simulink model "PMSM_EKF"  (R2014b)
settings: Solver=ode23tb  StartTime=0.0  StopTime=0.4  FixedStep=1e-6  RelTol=1e-4
libraries: powerlib x5, powerlib_extras x3, simulink x1
settings Model: Creator=guojinbo  LastModifiedBy=Lei
settings DataIOCC: SignalLoggingSaveFormat=ModelDataLogs
settings OptimizationCC: ExpressionDepthLimit=2147483647  InitFltsAndDblsToZero=on
settings DebuggingCC: UnderspecifiedInitializationDetection=Classic  MergeDetectMultiDrivingBlocksExec=none  FcnCallInpInsideContextMsg=UseLocalSettings  StateNameClashWarn=warning
settings GRTTargetCC: CombineOutputUpdateFcns=off  GRTInterface=on

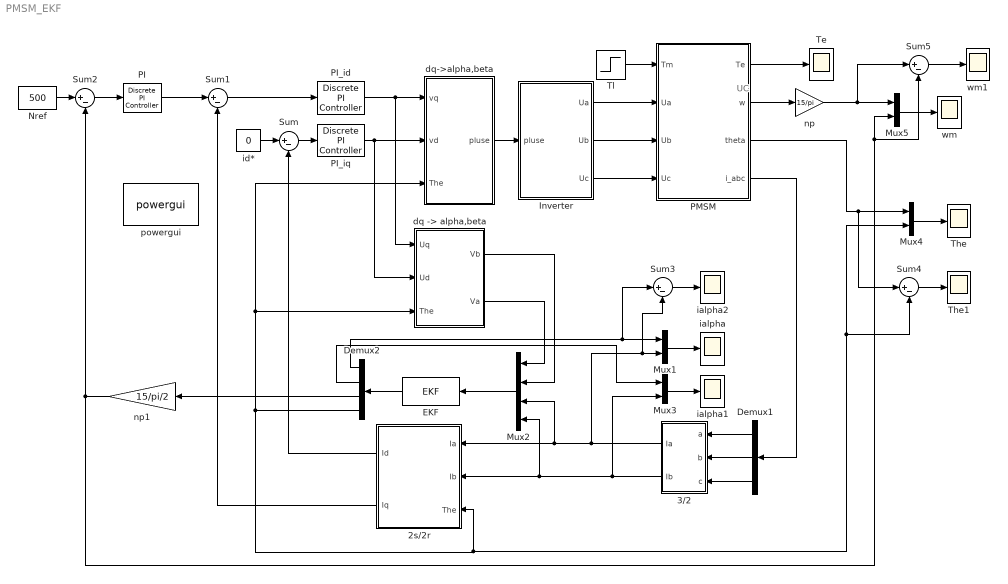
== system PMSM_EKF ==
  note: UC
  " PI " : powerlib_extras/Discrete  Control Blocks/Discrete PI Controller  Kp=0.6  Ki=0.8  Par_Limits=[40 -40]  Init=0  Ts=50e-6
  2s/2r : MATLAB Function  TreatAsAtomicUnit=on
  3/2 : MATLAB Function  TreatAsAtomicUnit=on
  Demux1 : Demux  Outputs=3
  Demux2 : Demux
  EKF : S-Function  FunctionName=EKF  EnableBusSupport=off
  Inverter : Subsystem
  Mux{1,3..5} (4 alike) : Mux  Inputs=2
  Mux2 : Mux
  Nref : Constant  Value=500
  PI_id : powerlib_extras/Discrete  Control Blocks/Discrete PI Controller  Kp=4.8  Ki=5.6  Par_Limits=[200 -200]  Init=0  Ts=50e-6
  PI_iq : powerlib_extras/Discrete  Control Blocks/Discrete PI Controller  Kp=8  Ki=9  Par_Limits=[200 -200]  Init=0  Ts=50e-6
  PMSM : Subsystem
  Sum{,1..5} (6 alike) : Sum  Inputs=|+-
  Te : Scope
      settings: YMin=486  YMax=500  SaveName=Te
  The : Scope
      settings: YMax=25  SaveName=The
  The1 : Scope
      settings: YMin=-0.5  YMax=1  SaveName=Thee
  Tl : Step  Time=0  Before=0.5  After=3.75  SampleTime=0
  "dq -> alpha,beta" : MATLAB Function  TreatAsAtomicUnit=on
  dq->alpha,beta : Subsystem
  ialpha : Scope
      settings: YMin=-100  YMax=600  SaveName=ialpha
  ialpha1 : Scope
      settings: YMin=-100  YMax=600  SaveName=ialpha1
  ialpha2 : Scope
      settings: YMin=-100  YMax=600  SaveName=ialpha2
  id* : Constant  Value=0
  np : Gain  Gain=15/pi
  np1 : Gain  Gain=15/pi/2
  powergui : powerlib/powergui  Priority=2  SimulationMode=Continuous  SolverType=Tustin/Backward Euler (TBE)  SampleTime=50e-6  frequency=60  SPID=off  DisableSnubberDevices=off  DisableRonSwitches=off  DisableVfSwitches=off  SwTol=0  DisplayEquations=off  Interpol=off  methode=off  Ts=0  frequencyindice=0  Pbase=100e6  ErrMax=1e-4  Iterations=50  UnitsV=kV  UnitsW=MW  FunctionMessages=off  echomessages=off  HookPort=off  EnableUseOfTLC=off  x0status=blocks  RestoreLinks=warning  ResistiveCurrentMeasurement=off  Frange=[0:2:500]  Ylog=off  Xlog=on  ShowGrid=off  save=off  variable=ZData  structure=0  ZoomFFT=on  StartTime=0.0  cycles=1  DisplayStyle=1  fundamental=60  FreqAxis=off  MaxFrequency=1000  frequencyindicesteady=1  RmsSteady=1  display=off
  wm : Scope
      settings: YMin=-100  YMax=600  SaveName=wm
  wm1 : Scope
      settings: YMin=-100  YMax=600  SaveName=wm1
  wires:
  PI_iq/1 -> "dq -> alpha,beta"/2(Ud), dq->alpha,beta/2(vd)
  Sum/1 -> PI_iq/1
  Sum1/1 -> PI_id/1
  id*/1 -> Sum/1
  Sum2/1 -> " PI "/1
  " PI "/1 -> Sum1/1
  PI_id/1 -> "dq -> alpha,beta"/1(Uq), dq->alpha,beta/1(vq)
  Nref/1 -> Sum2/1
  Tl/1 -> PMSM/1(Tm)
  PMSM/4(i_abc) -> Demux1/1
  PMSM/2(w) -> np/1
  Demux1/1 -> 3/2/1(a)
  Demux1/2 -> 3/2/2(b)
  Demux1/3 -> 3/2/3(c)
  3/2/1(Ia) -> Mux2/3, 2s/2r/1(Ia), Sum3/2, Mux1/2
  3/2/2(Ib) -> Mux2/4, 2s/2r/2(Ib), Mux3/2
  2s/2r/1(Id) -> Sum/2
  2s/2r/2(Iq) -> Sum1/2
  "dq -> alpha,beta"/2(Va) -> Mux2/1
  "dq -> alpha,beta"/1(Vb) -> Mux2/2
  Mux2/1 -> EKF/1
  EKF/1 -> Demux2/1
  Demux2/1 -> Sum3/1, Mux1/1
  Demux2/2 -> Mux3/1
  Demux2/3 -> np1/1
  Demux2/4 -> Sum4/2, Mux4/2, 2s/2r/3(The), dq->alpha,beta/3(The), "dq -> alpha,beta"/3(The)
  Inverter/1(Ua) -> PMSM/2(Ua)
  Inverter/2(Ub) -> PMSM/3(Ub)
  Inverter/3(Uc) -> PMSM/4(Uc)
  dq->alpha,beta/1(pluse) -> Inverter/1(pluse)
  PMSM/1(Te) -> Te/1
  PMSM/3(theta) -> Sum4/1, Mux4/1
  np/1 -> Sum5/1, Mux5/1
  Mux5/1 -> wm/1
  np1/1 -> Mux5/2, Sum5/2, Sum2/2
  Mux1/1 -> ialpha/1
  Sum4/1 -> The1/1
  Mux3/1 -> ialpha1/1
  Sum5/1 -> wm1/1
  Mux4/1 -> The/1
  Sum3/1 -> ialpha2/1

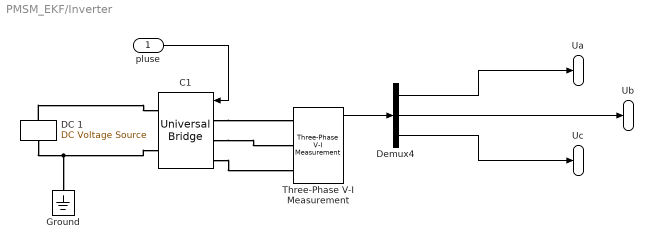
== system PMSM_EKF/Inverter ==
  pluse : Inport
  C1 : powerlib/Power Electronics/Universal Bridge  Arms=3  SnubberResistance=1e5  SnubberCapacitance=inf  Device=MOSFET / Diodes  Ron=1e-3  Lon=0  ForwardVoltages="[  0  0  ]"  ForwardVoltage=0  GTOparameters=[ 10e-6 , 20e-6 ]  IGBTparameters=[ 1e-6 , 2e-6 ]  Measurements=None  Measurements_2=None  converterType=Rectifier
  DC 1 : powerlib/Electrical Sources/DC Voltage Source  Amplitude=440  Measurements=None
  Demux4 : Demux  Outputs=3
  Ground : powerlib/Elements/Ground  LConnTagsString=a
  Three-Phase V-I Measurement : powerlib/Measurements/Three-Phase V-I Measurement  VoltageMeasurement=phase-to-ground  SetLabelV=off  LabelV=Vabc  Vpu=off  VpuLL=off  CurrentMeasurement=yes  SetLabelI=off  LabelI=Iabc  Ipu=off  Pbase=100e6  Vbase=500e3  OutputType=Complex  PhasorSimulation=off  PSBequivalent=0
  Ua : Outport
  Ub : Outport  Port=2
  Uc : Outport  Port=3
  wires:
  Three-Phase V-I Measurement/1 -> Demux4/1
  Demux4/1 -> Ua/1
  Demux4/2 -> Ub/1
  Demux4/3 -> Uc/1
  pluse/1 -> C1/1
  connections:
  DC 1/RConn1 -- C1/RConn1
  DC 1/LConn1 -- C1/RConn2 -- Ground/LConn1
  C1/LConn1 -- Three-Phase V-I Measurement/LConn1
  C1/LConn2 -- Three-Phase V-I Measurement/LConn2
  C1/LConn3 -- Three-Phase V-I Measurement/LConn3

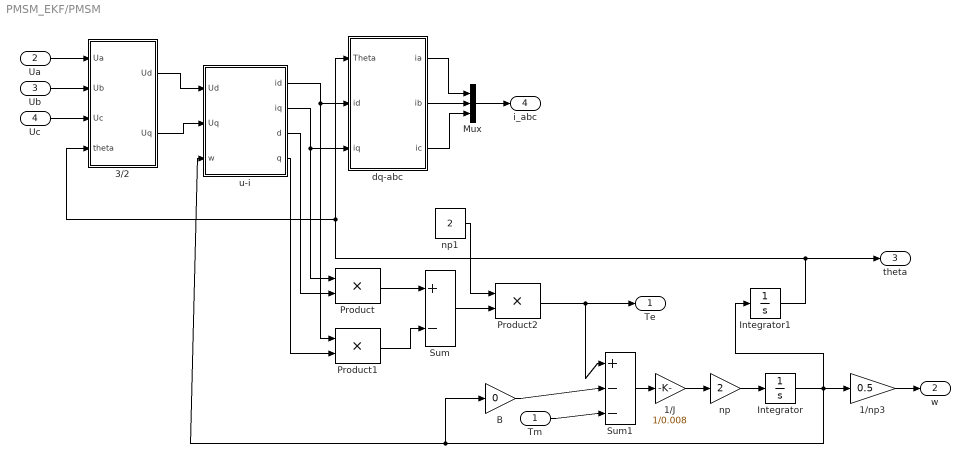
== system PMSM_EKF/PMSM ==
  Tm : Inport
  Ua : Inport  Port=2
  Ub : Inport  Port=3
  Uc : Inport  Port=4
  1/J : Gain  Gain=1/0.008  SaturateOnIntegerOverflow=on  OutDataTypeStr=Inherit: Same as input  ParamDataTypeStr=Inherit: Same as input
  1/np3 : Gain  Gain=0.5
  3/2 : Subsystem
  B : Gain  Gain=0  SaturateOnIntegerOverflow=on  OutDataTypeStr=Inherit: Same as input  ParamDataTypeStr=Inherit: Same as input
  Integrator : Integrator
  Integrator1 : Integrator
  Mux : Mux  Inputs=3
  Product : Product  SaturateOnIntegerOverflow=on  OutDataTypeStr=Inherit: Same as first input
  Product1 : Product  SaturateOnIntegerOverflow=on  OutDataTypeStr=Inherit: Same as first input
  Product2 : Product  SaturateOnIntegerOverflow=on  OutDataTypeStr=Inherit: Same as first input
  Sum : Sum  Inputs=+-  SaturateOnIntegerOverflow=on
  Sum1 : Sum  Inputs=|+--  SaturateOnIntegerOverflow=on
  dq-abc : Subsystem
  np : Gain  Gain=2
  np1 : Constant  Value=2
  u-i : Subsystem
  Te : Outport
  w : Outport  Port=2
  theta : Outport  Port=3
  i_abc : Outport  Port=4
  wires:
  u-i/1(id) -> dq-abc/2(id), Product1/1
  u-i/2(iq) -> dq-abc/3(iq), Product/1
  3/2/2(Uq) -> u-i/2(Uq)
  Product/1 -> Sum/1
  Product1/1 -> Sum/2
  Tm/1 -> Sum1/3
  B/1 -> Sum1/2
  Sum1/1 -> 1/J/1
  Integrator/1 -> Integrator1/1, 1/np3/1, u-i/3(w), B/1
  dq-abc/1(ia) -> Mux/1
  dq-abc/2(ib) -> Mux/2
  dq-abc/3(ic) -> Mux/3
  Mux/1 -> i_abc/1
  u-i/3(d) -> Product/2
  u-i/4(q) -> Product1/2
  np1/1 -> Product2/1
  Sum/1 -> Product2/2
  Product2/1 -> Sum1/1, Te/1
  1/J/1 -> np/1
  np/1 -> Integrator/1
  1/np3/1 -> w/1
  Integrator1/1 -> dq-abc/1(Theta), 3/2/4(theta), theta/1
  3/2/1(Ud) -> u-i/1(Ud)
  Ua/1 -> 3/2/1(Ua)
  Ub/1 -> 3/2/2(Ub)
  Uc/1 -> 3/2/3(Uc)

== system PMSM_EKF/dq->alpha,beta ==
  vq : Inport
  vd : Inport  Port=2
  The : Inport  Port=3
  Embedded MATLAB Function : MATLAB Function  TreatAsAtomicUnit=on
  Mux2 : Mux  Inputs=3
  SVPWM : Subsystem
  pluse : Outport
  wires:
  vd/1 -> Embedded MATLAB Function/2(Id)
  The/1 -> Embedded MATLAB Function/3(angle)
  vq/1 -> Embedded MATLAB Function/1(Iq)
  Embedded MATLAB Function/1(Vb) -> SVPWM/1(In1)
  Embedded MATLAB Function/2(Va) -> SVPWM/2(In2)
  SVPWM/2(chufab) -> Mux2/2
  SVPWM/3(chufac) -> Mux2/3
  SVPWM/1(chufa) -> Mux2/1
  Mux2/1 -> pluse/1

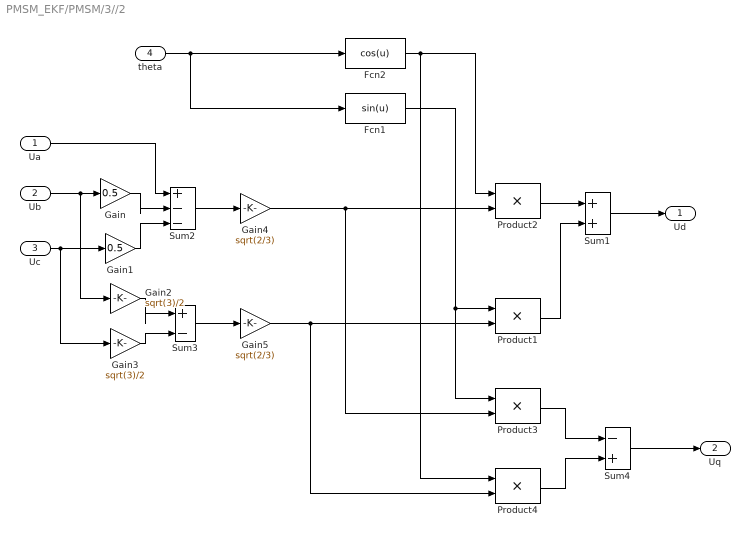
== system PMSM_EKF/PMSM/3//2 ==
  Ua : Inport
  Ub : Inport  Port=2
  Uc : Inport  Port=3
  theta : Inport  Port=4
  Fcn1 : Fcn  Expr=sin(u)
  Fcn2 : Fcn  Expr=cos(u)
  Gain : Gain  Gain=0.5
  Gain1 : Gain  Gain=0.5
  Gain2 : Gain  Gain=sqrt(3)/2
  Gain3 : Gain  Gain=sqrt(3)/2
  Gain4 : Gain  Gain=sqrt(2/3)
  Gain5 : Gain  Gain=sqrt(2/3)
  Product{1..4} (4 alike) : Product  SaturateOnIntegerOverflow=on  OutDataTypeStr=Inherit: Same as first input
  Sum1 : Sum
  Sum2 : Sum  Inputs=|+--
  Sum3 : Sum  Inputs=|+-
  Sum4 : Sum  Inputs=-+
  Ud : Outport
  Uq : Outport  Port=2
  wires:
  Ub/1 -> Gain/1, Gain2/1
  Sum2/1 -> Gain4/1
  Sum3/1 -> Gain5/1
  Ua/1 -> Sum2/1
  Gain2/1 -> Sum3/1
  Gain3/1 -> Sum3/2
  Gain/1 -> Sum2/2
  Gain1/1 -> Sum2/3
  Gain4/1 -> Product2/2, Product3/2
  Gain5/1 -> Product1/2, Product4/2
  Uc/1 -> Gain1/1, Gain3/1
  theta/1 -> Fcn2/1, Fcn1/1
  Fcn2/1 -> Product2/1, Product4/1
  Fcn1/1 -> Product1/1, Product3/1
  Product2/1 -> Sum1/1
  Product1/1 -> Sum1/2
  Sum1/1 -> Ud/1
  Product3/1 -> Sum4/1
  Product4/1 -> Sum4/2
  Sum4/1 -> Uq/1

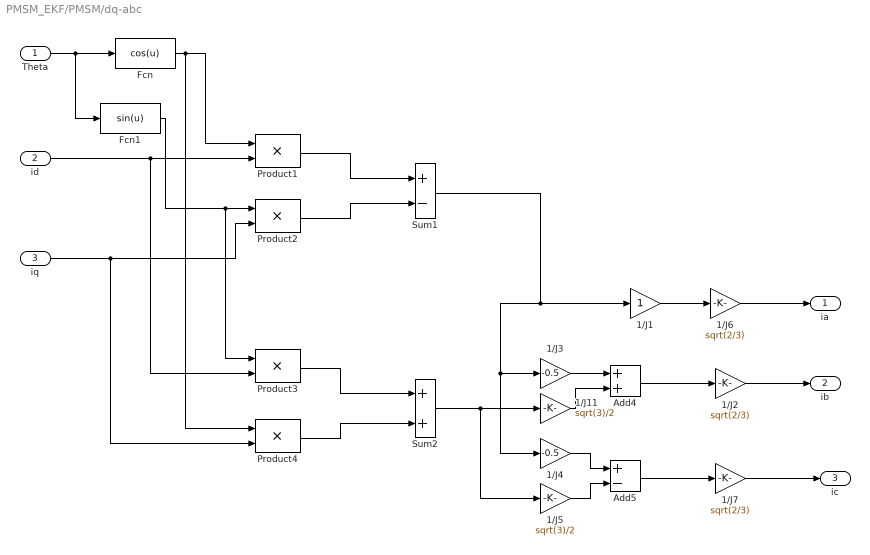
== system PMSM_EKF/PMSM/dq-abc ==
  Theta : Inport
  id : Inport  Port=2
  iq : Inport  Port=3
  1/J1 : Gain
  1/J11 : Gain  Gain=sqrt(3)/2
  1/J2 : Gain  Gain=sqrt(2/3)
  1/J3 : Gain  Gain=-0.5
  1/J4 : Gain  Gain=-0.5
  1/J5 : Gain  Gain=sqrt(3)/2
  1/J6 : Gain  Gain=sqrt(2/3)
  1/J7 : Gain  Gain=sqrt(2/3)
  Add4 : Sum
  Add5 : Sum  Inputs=+-
  Fcn : Fcn  Expr=cos(u)
  Fcn1 : Fcn  Expr=sin(u)
  Product{1..4} (4 alike) : Product  SaturateOnIntegerOverflow=on  OutDataTypeStr=Inherit: Same as first input
  Sum1 : Sum  Inputs=+-  SaturateOnIntegerOverflow=on
  Sum2 : Sum  SaturateOnIntegerOverflow=on
  ia : Outport
  ib : Outport  Port=2
  ic : Outport  Port=3
  wires:
  Theta/1 -> Fcn/1, Fcn1/1
  Fcn/1 -> Product1/1, Product4/1
  id/1 -> Product1/2, Product3/2
  Fcn1/1 -> Product3/1, Product2/1
  iq/1 -> Product2/2, Product4/2
  Product1/1 -> Sum1/1
  Product2/1 -> Sum1/2
  Product3/1 -> Sum2/1
  Product4/1 -> Sum2/2
  Sum1/1 -> 1/J3/1, 1/J4/1, 1/J1/1
  Sum2/1 -> 1/J11/1, 1/J5/1
  1/J1/1 -> 1/J6/1
  1/J3/1 -> Add4/1
  1/J11/1 -> Add4/2
  1/J4/1 -> Add5/1
  1/J5/1 -> Add5/2
  Add4/1 -> 1/J2/1
  Add5/1 -> 1/J7/1
  1/J6/1 -> ia/1
  1/J2/1 -> ib/1
  1/J7/1 -> ic/1

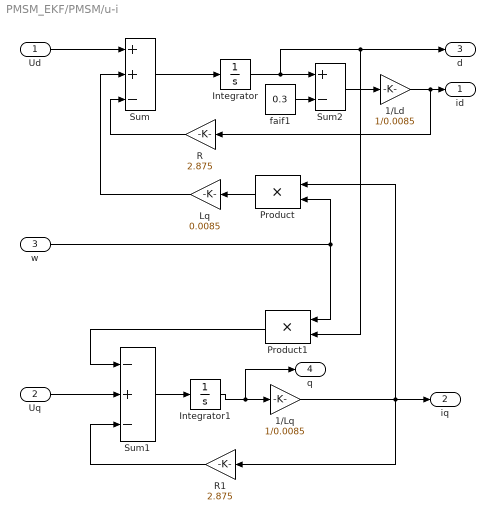
== system PMSM_EKF/PMSM/u-i ==
  Ud : Inport
  Uq : Inport  Port=2
  w : Inport  Port=3
  1/Ld : Gain  Gain=1/0.0085  SaturateOnIntegerOverflow=on  OutDataTypeStr=Inherit: Same as input  ParamDataTypeStr=Inherit: Same as input
  1/Lq : Gain  Gain=1/0.0085  SaturateOnIntegerOverflow=on  OutDataTypeStr=Inherit: Same as input  ParamDataTypeStr=Inherit: Same as input
  Integrator : Integrator  InitialCondition=0.01
  Integrator1 : Integrator
  Lq : Gain  Gain=0.0085  SaturateOnIntegerOverflow=on  OutDataTypeStr=Inherit: Same as input  ParamDataTypeStr=Inherit: Same as input
  Product : Product  SaturateOnIntegerOverflow=on  OutDataTypeStr=Inherit: Same as first input
  Product1 : Product  SaturateOnIntegerOverflow=on  OutDataTypeStr=Inherit: Same as first input
  R : Gain  Gain=2.875  SaturateOnIntegerOverflow=on  OutDataTypeStr=Inherit: Same as input  ParamDataTypeStr=Inherit: Same as input
  R1 : Gain  Gain=2.875  SaturateOnIntegerOverflow=on  OutDataTypeStr=Inherit: Same as input  ParamDataTypeStr=Inherit: Same as input
  Sum : Sum  Inputs=++-  SaturateOnIntegerOverflow=on
  Sum1 : Sum  Inputs=-+-  SaturateOnIntegerOverflow=on
  Sum2 : Sum  Inputs=+-  SaturateOnIntegerOverflow=on
  faif1 : Constant  Value=0.3
  id : Outport
  iq : Outport  Port=2
  d : Outport  Port=3
  q : Outport  Port=4
  wires:
  Ud/1 -> Sum/1
  Sum/1 -> Integrator/1
  Product/1 -> Lq/1
  Lq/1 -> Sum/2
  w/1 -> Product1/1, Product/2
  R/1 -> Sum/3
  R1/1 -> Sum1/3
  Sum1/1 -> Integrator1/1
  Product1/1 -> Sum1/1
  Integrator/1 -> Sum2/1, Product1/2, d/1
  faif1/1 -> Sum2/2
  Sum2/1 -> 1/Ld/1
  1/Ld/1 -> id/1, R/1
  Uq/1 -> Sum1/2
  Integrator1/1 -> 1/Lq/1, q/1
  1/Lq/1 -> iq/1, Product/1, R1/1

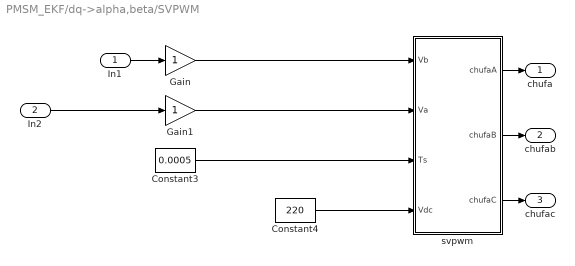
== system PMSM_EKF/dq->alpha,beta/SVPWM ==
  In1 : Inport
  In2 : Inport  Port=2
  Constant3 : Constant  Value=0.0005
  Constant4 : Constant  Value=220
  Gain : Gain
  Gain1 : Gain
  svpwm : Subsystem
  chufa : Outport
  chufab : Outport  Port=2
  chufac : Outport  Port=3
  wires:
  Constant3/1 -> svpwm/3(Ts)
  Constant4/1 -> svpwm/4(Vdc)
  svpwm/1(chufaA) -> chufa/1
  Gain/1 -> svpwm/1(Vb)
  In2/1 -> Gain1/1
  Gain1/1 -> svpwm/2(Va)
  In1/1 -> Gain/1
  svpwm/3(chufaC) -> chufac/1
  svpwm/2(chufaB) -> chufab/1

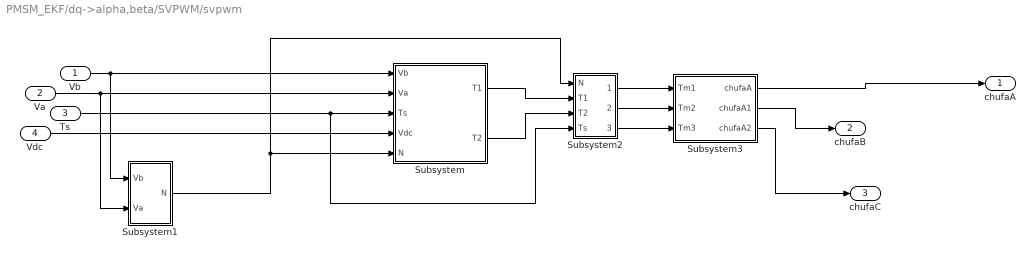
== system PMSM_EKF/dq->alpha,beta/SVPWM/svpwm ==
  Vb : Inport
  Va : Inport  Port=2
  Ts : Inport  Port=3
  Vdc : Inport  Port=4
  Subsystem : Subsystem
  Subsystem1 : Subsystem
  Subsystem2 : Subsystem
  Subsystem3 : Subsystem
  chufaA : Outport
  chufaB : Outport  Port=2
  chufaC : Outport  Port=3
  wires:
  Vb/1 -> Subsystem1/1(Vb), Subsystem/1(Vb)
  Va/1 -> Subsystem1/2(Va), Subsystem/2(Va)
  Ts/1 -> Subsystem/3(Ts), Subsystem2/4(Ts)
  Vdc/1 -> Subsystem/4(Vdc)
  Subsystem1/1(N) -> Subsystem/5(N), Subsystem2/1(N)
  Subsystem/1(T1) -> Subsystem2/2(T1)
  Subsystem/2(T2) -> Subsystem2/3(T2)
  Subsystem2/1(Tm1) -> Subsystem3/1(Tm1)
  Subsystem2/2(Tm2) -> Subsystem3/2(Tm2)
  Subsystem2/3(Tm3) -> Subsystem3/3(Tm3)
  Subsystem3/1(chufaA) -> chufaA/1
  Subsystem3/2(chufaA1) -> chufaB/1
  Subsystem3/3(chufaA2) -> chufaC/1

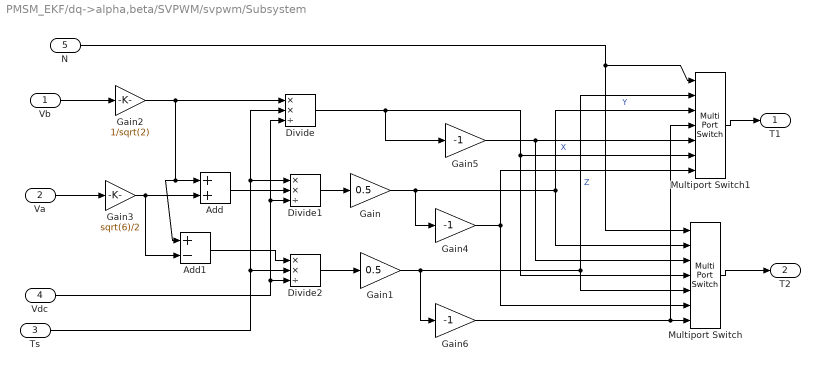
== system PMSM_EKF/dq->alpha,beta/SVPWM/svpwm/Subsystem ==
  Vb : Inport
  Va : Inport  Port=2
  Ts : Inport  Port=3
  Vdc : Inport  Port=4
  N : Inport  Port=5
  Add : Sum
  Add1 : Sum  Inputs=+-
  Divide : Product  Inputs=**/
  Divide1 : Product  Inputs=**/
  Divide2 : Product  Inputs=**/
  Gain : Gain  Gain=0.5
  Gain1 : Gain  Gain=0.5
  Gain2 : Gain  Gain=1/sqrt(2)
  Gain3 : Gain  Gain=sqrt(6)/2
  Gain4 : Gain  Gain=-1
  Gain5 : Gain  Gain=-1
  Gain6 : Gain  Gain=-1
  Multiport Switch : MultiPortSwitch  Inputs=6
  Multiport Switch1 : MultiPortSwitch  Inputs=6
  T1 : Outport
  T2 : Outport  Port=2
  wires:
  Vb/1 -> Gain2/1
  Gain2/1 -> Divide/1, Add/1, Add1/1
  Divide/1 -> Gain5/1, Multiport Switch1/6, Multiport Switch/4  "X"
  Va/1 -> Gain3/1
  Gain3/1 -> Add/2, Add1/2
  Gain/1 -> Gain4/1, Multiport Switch/2, Multiport Switch1/3  "Y"
  Gain1/1 -> Gain6/1, Multiport Switch1/2, Multiport Switch/5  "Z"
  Divide1/1 -> Gain/1
  Divide2/1 -> Gain1/1
  Vdc/1 -> Divide2/3, Divide1/3, Divide/3
  Ts/1 -> Divide2/2, Divide1/1, Divide/2
  Add/1 -> Divide1/2
  Add1/1 -> Divide2/1
  N/1 -> Multiport Switch1/1, Multiport Switch/1
  Multiport Switch/1 -> T2/1
  Multiport Switch1/1 -> T1/1
  Gain5/1 -> Multiport Switch1/5, Multiport Switch/3
  Gain4/1 -> Multiport Switch/6, Multiport Switch1/7
  Gain6/1 -> Multiport Switch1/4, Multiport Switch/7

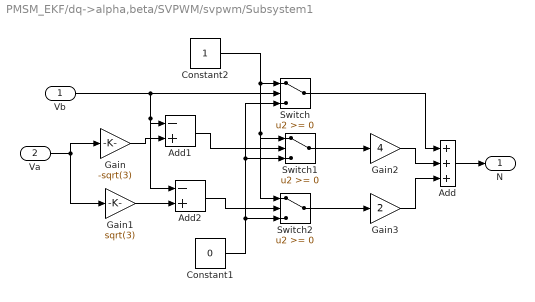
== system PMSM_EKF/dq->alpha,beta/SVPWM/svpwm/Subsystem1 ==
  Vb : Inport
  Va : Inport  Port=2
  Add : Sum  Inputs=+++
  Add1 : Sum  Inputs=-+
  Add2 : Sum  Inputs=-+
  Constant1 : Constant  Value=0
  Constant2 : Constant
  Gain : Gain  Gain=-sqrt(3)
  Gain1 : Gain  Gain=sqrt(3)
  Gain2 : Gain  Gain=4
  Gain3 : Gain  Gain=2
  Switch : Switch
  Switch1 : Switch
  Switch2 : Switch
  N : Outport
  wires:
  Add1/1 -> Switch1/2
  Add2/1 -> Switch2/2
  Gain1/1 -> Add2/2
  Gain/1 -> Add1/2
  Va/1 -> Gain/1, Gain1/1
  Vb/1 -> Switch/2, Add1/1, Add2/1
  Constant2/1 -> Switch/1, Switch1/1, Switch2/1
  Constant1/1 -> Switch2/3, Switch1/3, Switch/3
  Switch2/1 -> Gain3/1
  Switch1/1 -> Gain2/1
  Switch/1 -> Add/1
  Gain3/1 -> Add/3
  Gain2/1 -> Add/2
  Add/1 -> N/1

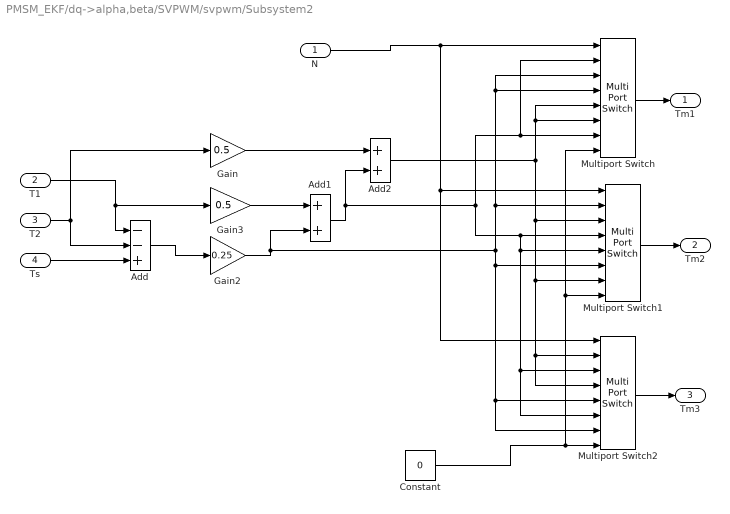
== system PMSM_EKF/dq->alpha,beta/SVPWM/svpwm/Subsystem2 ==
  N : Inport
  T1 : Inport  Port=2
  T2 : Inport  Port=3
  Ts : Inport  Port=4
  Add : Sum  Inputs=--+
  Add1 : Sum
  Add2 : Sum
  Constant : Constant  Value=0
  Gain : Gain  Gain=0.5
  Gain2 : Gain  Gain=0.25
  Gain3 : Gain  Gain=0.5
  Multiport Switch : MultiPortSwitch  Inputs=7
  Multiport Switch1 : MultiPortSwitch  Inputs=7
  Multiport Switch2 : MultiPortSwitch  Inputs=7
  Tm1 : Outport
  Tm2 : Outport  Port=2
  Tm3 : Outport  Port=3
  wires:
  T1/1 -> Gain3/1, Add/1
  T2/1 -> Gain/1, Add/2
  Ts/1 -> Add/3
  Add/1 -> Gain2/1
  N/1 -> Multiport Switch/1, Multiport Switch1/1, Multiport Switch2/1
  Gain3/1 -> Add1/1
  Gain2/1 -> Add1/2, Multiport Switch/3, Multiport Switch/4, Multiport Switch1/2, Multiport Switch1/6, Multiport Switch2/7, Multiport Switch2/5
  Gain/1 -> Add2/1
  Add1/1 -> Add2/2, Multiport Switch/2, Multiport Switch/7, Multiport Switch1/4, Multiport Switch1/5, Multiport Switch2/3, Multiport Switch2/6
  Add2/1 -> Multiport Switch/6, Multiport Switch/5, Multiport Switch1/3, Multiport Switch1/7, Multiport Switch2/2, Multiport Switch2/4
  Constant/1 -> Multiport Switch2/8, Multiport Switch/8, Multiport Switch1/8
  Multiport Switch2/1 -> Tm3/1
  Multiport Switch1/1 -> Tm2/1
  Multiport Switch/1 -> Tm1/1

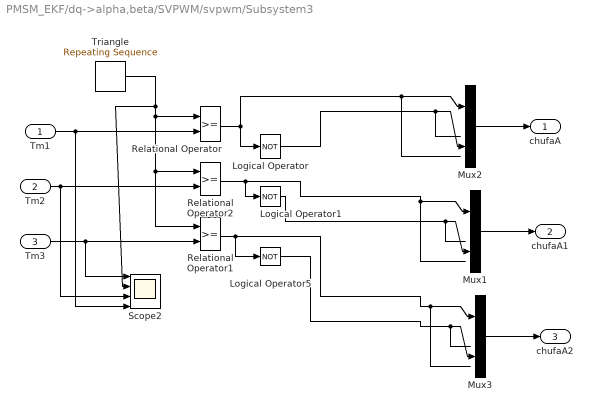
== system PMSM_EKF/dq->alpha,beta/SVPWM/svpwm/Subsystem3 ==
  Tm1 : Inport
  Tm2 : Inport  Port=2
  Tm3 : Inport  Port=3
  Logical Operator : Logic  Operator=NOT  OutDataTypeStr=float('double')
  Logical Operator1 : Logic  Operator=NOT  OutDataTypeStr=float('double')
  Logical Operator5 : Logic  Operator=NOT  OutDataTypeStr=float('double')
  Mux1 : Mux  Inputs=2
  Mux2 : Mux  Inputs=2
  Mux3 : Mux  Inputs=2
  Relational Operator : RelationalOperator  OutDataTypeStr=float('double')  InputSameDT=on
  Relational Operator1 : RelationalOperator  OutDataTypeStr=float('double')  InputSameDT=on
  Relational Operator2 : RelationalOperator  OutDataTypeStr=float('double')  InputSameDT=on
  Scope2 : Scope  NumInputPorts=4
      settings: TickLabels=on  TimeRange=0.0002904125448409678  YMin=2.4745e-005~0~2.556e-005~2.52505e-005  YMax=2.47495e-005~5e-005~2.5569e-005~2.5255e-005  SaveName=ScopeData5  Decimation=1000  SampleInput=on
  Triangle : simulink/Sources/Repeating Sequence  rep_seq_t=[0 0.00025 0.0005]  rep_seq_y=[0 0.00025 0]
  chufaA : Outport
  chufaA1 : Outport  Port=2
  chufaA2 : Outport  Port=3
  wires:
  Triangle/1 -> Relational Operator/1, Relational Operator1/1, Relational Operator2/1, Scope2/2
  Tm1/1 -> Relational Operator/2, Scope2/4
  Tm2/1 -> Relational Operator2/2, Scope2/3
  Tm3/1 -> Relational Operator1/2, Scope2/1
  Relational Operator/1 -> Logical Operator/1, Mux2/1
  Relational Operator2/1 -> Logical Operator1/1, Mux1/1
  Relational Operator1/1 -> Logical Operator5/1, Mux3/1
  Logical Operator1/1 -> Mux1/2
  Logical Operator5/1 -> Mux3/2
  Logical Operator/1 -> Mux2/2
  Mux2/1 -> chufaA/1
  Mux1/1 -> chufaA1/1
  Mux3/1 -> chufaA2/1

== matlab function PMSM_EKF/dq -> alpha,beta ==
  data: Uq input; Vb output; Ud input; Va output; The input
function [Vb,Va] = fcn(Uq,Ud,The)
% This block supports an embeddable subset of the MATLAB language.
% See the help menu for details. 


Vb=Uq*cos(The)+Ud*sin(The);
Va=Ud*cos(The)-Uq*sin(The);

== matlab function PMSM_EKF/dq->alpha,beta/Embedded MATLAB Function ==
  data: Iq input; Vb output; Id input; Va output; angle input
function [Vb,Va] = fcn(Iq,Id,angle)
% This block supports an embeddable subset of the MATLAB language.
% See the help menu for details. 


Vb=Iq*cos(angle)+Id*sin(angle);
Va=Id*cos(angle)-Iq*sin(angle);

== matlab function PMSM_EKF/3/2 ==
  data: Ia output; a input; b input; Ib output; c input
function [Ia,Ib] = fcn(a,b,c)
% This block supports an embeddable subset of the MATLAB language.
% See the help menu for details. 


Ib=(b-c)*0.707;%/sqrt(3);
Ia=(2*a-b-c)*0.4082;%/3;

== matlab function PMSM_EKF/2s/2r ==
  data: Ia input; Ib input; Id output; Iq output; The input
function [Id,Iq] = fcn(Ia,Ib,The)
% This block supports an embeddable subset of the MATLAB language.
% See the help menu for details. 


Id=Ia*cos(The)+Ib*sin(The);
Iq=Ib*cos(The)-Ia*sin(The);
